simulink model "calculate_filter_coefficients_sim"  (R2020b)
settings: Solver=FixedStepAuto  StartTime=0.0  StopTime=stopTime  RelTol=1e-3
InitFcn:
  | initCallback
StopFcn:
  | stopCallback
values from neighbouring files (symbols this model uses):
  fs = 48e3    (= 48000)    [modelparameters.m]
settings Model: Creator=t96f346  LastModifiedBy=conno
settings DataIOCC: ReturnWorkspaceOutputs=off

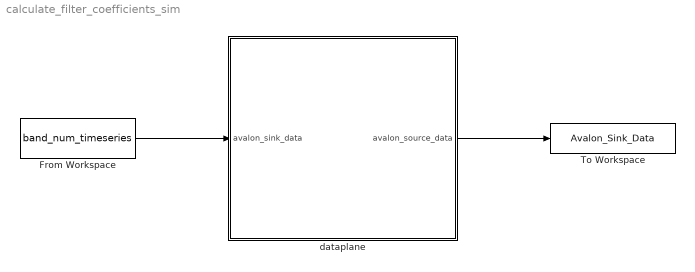
== system calculate_filter_coefficients_sim ==
  From Workspace : FromWorkspace  VariableName=band_num_timeseries  SampleTime=1/fs
  To Workspace : ToWorkspace  VariableName=Avalon_Sink_Data  SampleTime=-1
  dataplane : Subsystem  TreatAsAtomicUnit=on
  wires:
  From Workspace/1 -> dataplane/1(avalon_sink_data)
  dataplane/1(avalon_source_data) -> To Workspace/1

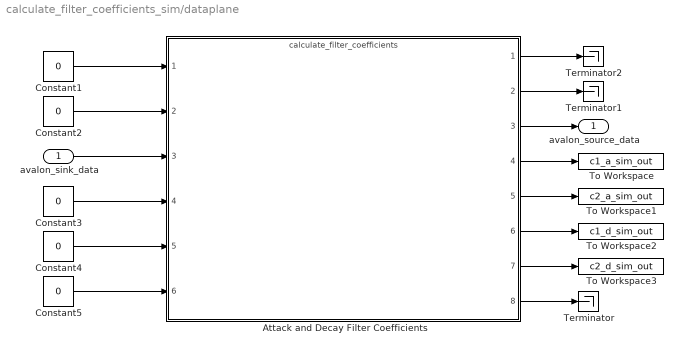
== system calculate_filter_coefficients_sim/dataplane ==
  avalon_sink_data : Inport
  Attack and Decay Filter Coefficients : ModelReference  ModelNameDialog=calculate_filter_coefficients.slx  SimulationMode=Normal  ModelReferenceVersion=2.45
  Constant1 : Constant  Value=0  OutDataTypeStr=boolean  SampleTime=-1
  Constant2 : Constant  Value=0  OutDataTypeStr=fixdt(1,40,32)  SampleTime=-1
  Constant3 : Constant  Value=0  OutDataTypeStr=fixdt(0,16,16)  SampleTime=-1
  Constant4 : Constant  Value=0  OutDataTypeStr=uint8  SampleTime=-1
  Constant5 : Constant  Value=0  OutDataTypeStr=boolean  SampleTime=-1
  Terminator : Terminator
  Terminator1 : Terminator
  Terminator2 : Terminator
  To Workspace : ToWorkspace  VariableName=c1_a_sim_out  SampleTime=-1
  To Workspace1 : ToWorkspace  VariableName=c2_a_sim_out  SampleTime=-1
  To Workspace2 : ToWorkspace  VariableName=c1_d_sim_out  SampleTime=-1
  To Workspace3 : ToWorkspace  VariableName=c2_d_sim_out  SampleTime=-1
  avalon_source_data : Outport  VectorParamsAs1DForOutWhenUnconnected=off
  wires:
  avalon_sink_data/1 -> Attack and Decay Filter Coefficients/3
  Attack and Decay Filter Coefficients/3 -> avalon_source_data/1
  Attack and Decay Filter Coefficients/4 -> To Workspace/1
  Attack and Decay Filter Coefficients/5 -> To Workspace1/1
  Attack and Decay Filter Coefficients/6 -> To Workspace2/1
  Attack and Decay Filter Coefficients/7 -> To Workspace3/1
  Attack and Decay Filter Coefficients/8 -> Terminator/1
  Attack and Decay Filter Coefficients/2 -> Terminator1/1
  Attack and Decay Filter Coefficients/1 -> Terminator2/1
  Constant1/1 -> Attack and Decay Filter Coefficients/1
  Constant2/1 -> Attack and Decay Filter Coefficients/2
  Constant4/1 -> Attack and Decay Filter Coefficients/5
  Constant3/1 -> Attack and Decay Filter Coefficients/4
  Constant5/1 -> Attack and Decay Filter Coefficients/6
